simulink model "proiect_ZieglerNichols"  (R2022b)
settings: Solver=VariableStepAuto  StartTime=0.0  StopTime=1000.0  RelTol=1e-3
settings Model: Creator=ALex  LastModifiedBy=ALex
settings DataIOCC: ReturnWorkspaceOutputs=off

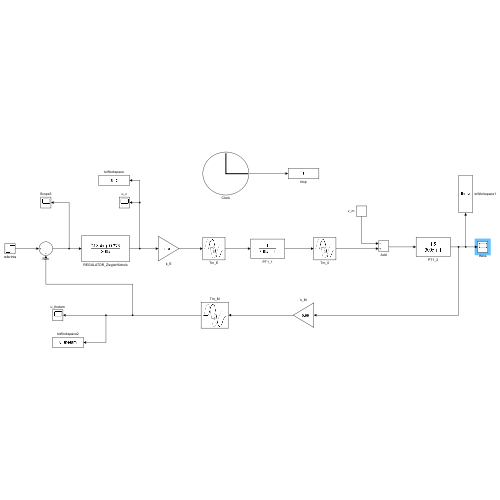
[thumbnail: Simulink's stored preview of the top-level diagram]
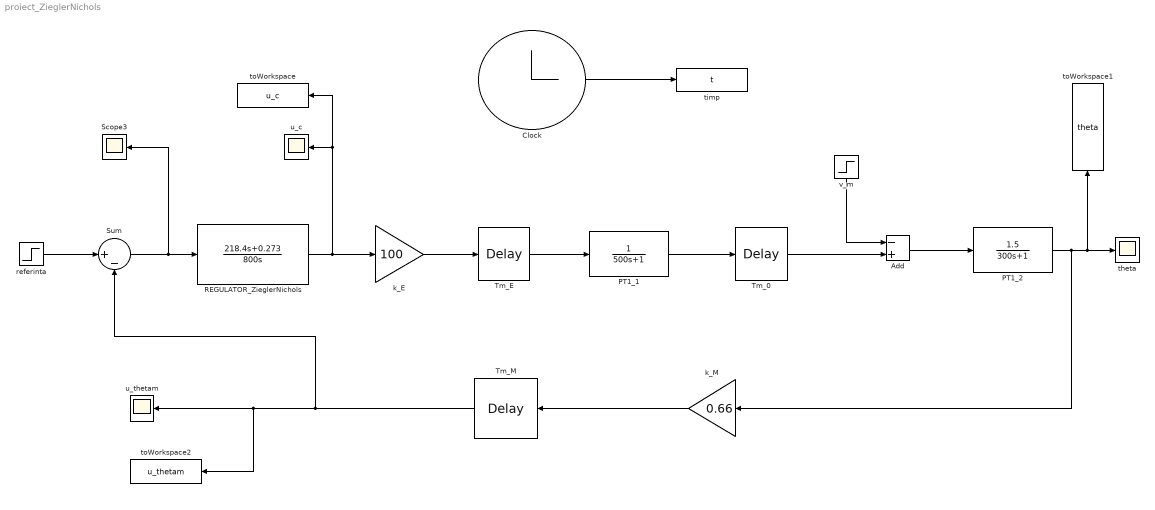
== system proiect_ZieglerNichols ==
  Add : Sum  Inputs=-+
  Clock : Clock
  PT1_1 : TransferFcn  Denominator=[500 1]
  PT1_2 : TransferFcn  Numerator=[1.5]  Denominator=[300 1]
  REGULATOR_ZieglerNichols : TransferFcn  Numerator=[218.4 0.273]  Denominator=[800 0]
  Scope3 : Scope
  Sum : Sum  Inputs=|+-
  Tm_0 : TransportDelay  DelayTime=125
  Tm_E : TransportDelay  DelayTime=5
  Tm_M : TransportDelay  DelayTime=20
  k_E : Gain  Gain=100
  k_M : Gain  Gain=0.66
  referinta : Step  Time=0  After=650  SampleTime=0
  theta : Scope
  timp : ToWorkspace  VariableName=t  SampleTime=-1
  toWorkspace : ToWorkspace  VariableName=u_c  SampleTime=-1
  toWorkspace1 : ToWorkspace  VariableName=theta  SampleTime=-1
  toWorkspace2 : ToWorkspace  VariableName=u_thetam  SampleTime=-1
  u_c : Scope
  u_thetam : Scope
  v_m : Step  Time=20000  After=50  SampleTime=0
  wires:
  Clock/1 -> timp/1
  v_m/1 -> Add/1
  REGULATOR_ZieglerNichols/1 -> toWorkspace/1, u_c/1, k_E/1
  PT1_2/1 -> k_M/1, theta/1, toWorkspace1/1
  Tm_0/1 -> Add/2
  Tm_M/1 -> Sum/2, toWorkspace2/1, u_thetam/1
  referinta/1 -> Sum/1
  Sum/1 -> Scope3/1, REGULATOR_ZieglerNichols/1
  PT1_1/1 -> Tm_0/1
  k_M/1 -> Tm_M/1
  Add/1 -> PT1_2/1
  k_E/1 -> Tm_E/1
  Tm_E/1 -> PT1_1/1
